simulink model "Readdata_Model"  (R2024b)
settings: Solver=VariableStepAuto  StartTime=0.0  StopTime=10.0  RelTol=1e-3
libraries: NSA_DEVS_LOGISTICS x5, NSA_DEVS_SINKS x3, NSA_DEVS_SOURCES x1
settings Model: Creator=david  LastModifiedBy=peter
settings RTWCC: GPUComputeCapability=3.5

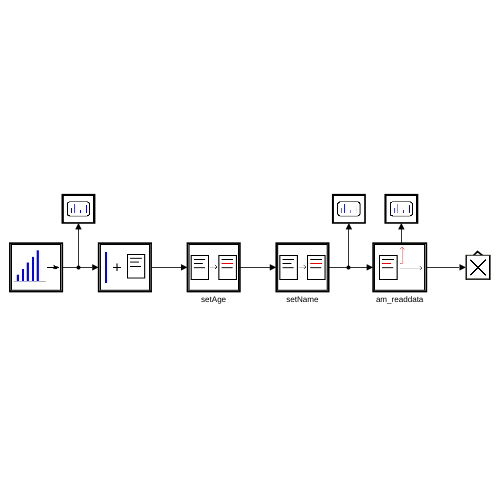
[thumbnail: Simulink's stored preview of the top-level diagram]
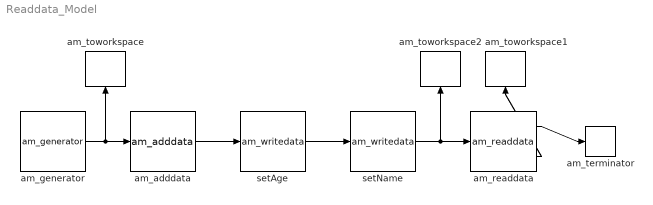
== system Readdata_Model ==
  am_adddata : NSA_DEVS_LOGISTICS/am_adddata  fields="[\"age\", \"name\"]"  values="[\"36\", \"Peter\"]"  numeric=[true, false]  infield="\"id\""  tau=[0,1]  debug=0
      settings: SourceProductName=Logistics
  am_generator : NSA_DEVS_SOURCES/am_generator  tG=1  n0=1  nG=6  tD=[0,2]  debug=0
      settings: SourceProductName=Sources
  am_readdata : NSA_DEVS_LOGISTICS/am_readdata  field="\"age\""  tau=[0,1]  debug=0
      settings: SourceProductName=Logistics
  am_terminator : NSA_DEVS_LOGISTICS/am_terminator  tau=[0,1]  debug=0
      settings: SourceProductName=Logistics
  am_toworkspace : NSA_DEVS_SINKS/am_toworkspace  varname="\"genOut\""  t0=0  format="\"vector\""  tau=[0,3]  debug=0
      settings: SourceProductName=Sinks
  am_toworkspace1 : NSA_DEVS_SINKS/am_toworkspace  varname="\"valOut\""  t0=0  format="\"vector\""  tau=[0,3]  debug=0
      settings: SourceProductName=Sinks
  am_toworkspace2 : NSA_DEVS_SINKS/am_toworkspace  varname="\"dataOut\""  t0=0  format="\"vector\""  tau=[0,3]  debug=0
      settings: SourceProductName=Sinks
  setAge : NSA_DEVS_LOGISTICS/am_writedata  inFields="[\"age\", \"id\"]"  outField="\"age\""  changeFunc="\"out = in(1) + in(2);\""  tau=[0,1]  debug=0
      settings: SourceProductName=Logistics
  setName : NSA_DEVS_LOGISTICS/am_writedata  inFields="[\"name\", \"age\"]"  outField="\"name\""  changeFunc="\"out = in(1) + in(2);\""  tau=[0,1]  debug=0
      settings: SourceProductName=Logistics
  wires:
  am_generator/1 -> am_adddata/1, am_toworkspace/1
  am_adddata/1 -> setAge/1
  setAge/1 -> setName/1
  am_readdata/1 -> am_terminator/1
  am_readdata/2 -> am_toworkspace1/1
  setName/1 -> am_readdata/1, am_toworkspace2/1
